simulink model "nedc_cycle"  (R2014b)
settings: Solver=ode3  StartTime=0.0  StopTime=1180  FixedStep=0.001  RelTol=1e-3
values from neighbouring files (symbols this model uses):
  a_nedc = [0;nedc.acceleration]    [nedc_data.m]
  a_sample = [a_sample; a_sample(end)]    [nedc_data.m]
  t_nedc = [0;cumsum(duration_nedc)]    [nedc_data.m]
  t_sample = [0; t_sample]    [nedc_data.m]
settings Model: Creator=uisee  LastModifiedBy=uisee

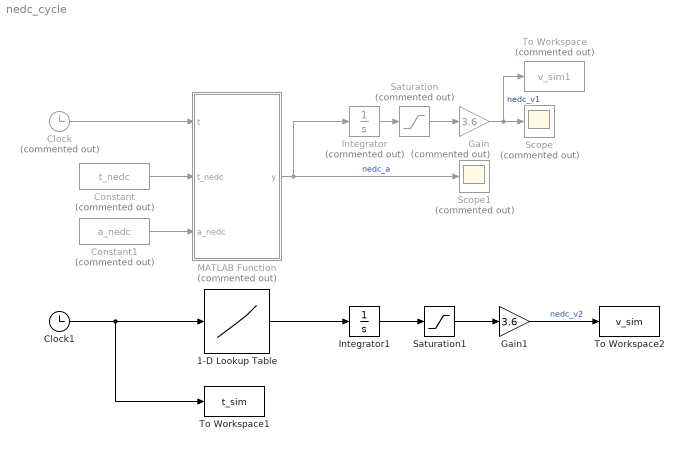
== system nedc_cycle ==
  1-D Lookup Table : Lookup_n-D  NumberOfTableDimensions=1  BreakpointsForDimension1=t_sample  Table=a_sample  InternalRulePriority=Speed  RndMeth=Simplest  InputSameDT=on
  Clock : Clock  Commented=on
  Clock1 : Clock
  Constant : Constant  Commented=on  Value=t_nedc
  Constant1 : Constant  Commented=on  Value=a_nedc
  Gain : Gain  Commented=on  Gain=3.6
  Gain1 : Gain  Gain=3.6
  Integrator : Integrator  Commented=on
  Integrator1 : Integrator
  MATLAB Function : MATLAB Function  Commented=on  TreatAsAtomicUnit=on
  Saturation : Saturate  Commented=on  UpperLimit=200  LowerLimit=0
  Saturation1 : Saturate  UpperLimit=200  LowerLimit=0
  Scope : Scope  Commented=on
  Scope1 : Scope  Commented=on
  To Workspace : ToWorkspace  Commented=on  VariableName=v_sim1  SampleTime=-1
      settings: Decimation=3
  To Workspace1 : ToWorkspace  VariableName=t_sim  SampleTime=-1
      settings: Decimation=3
  To Workspace2 : ToWorkspace  VariableName=v_sim  SampleTime=-1
      settings: Decimation=3
  wires:
  Clock/1 -> MATLAB Function/1(t)
  MATLAB Function/1(y) -> Integrator/1, Scope1/1  "nedc_a"
  Integrator/1 -> Saturation/1
  Gain/1 -> To Workspace/1, Scope/1  "nedc_v1"
  Constant/1 -> MATLAB Function/2(t_nedc)
  Constant1/1 -> MATLAB Function/3(a_nedc)
  Saturation/1 -> Gain/1
  1-D Lookup Table/1 -> Integrator1/1
  Integrator1/1 -> Saturation1/1
  Gain1/1 -> To Workspace2/1  "nedc_v2"
  Saturation1/1 -> Gain1/1
  Clock1/1 -> To Workspace1/1, 1-D Lookup Table/1

== matlab function nedc_cycle/MATLAB Function ==
  data: t input; y output; t_nedc input; a_nedc input
function y = look_up(t, t_nedc, a_nedc)
%#codegen
a = acceleration_vs_time(t, t_nedc, a_nedc);
y = a;
